simulink model "PartA"  (R2022b)
settings: Solver=VariableStepAuto  StartTime=0.0  StopTime=0.2  RelTol=1e-3
values from neighbouring files (symbols this model uses):
  Freq = 60    [main.mat]    (also in main1.m)
  Lload = 0.01    [main.mat]    (also in main1.m)
  Rload = 2    [main.mat]    (also in main1.m)
  Vdc = 250    [main.mat]    (also in main1.m)
libraries: spspowerguiLib x1
settings Model: Creator=pouyaalaei  LastModifiedBy=igho
settings SolverCC: AlgebraicLoopSolver=TrustRegion
settings DataIOCC: ReturnWorkspaceOutputs=off
settings DebuggingCC: UnconnectedInputMsg=warning  UnconnectedOutputMsg=warning  UnconnectedLineMsg=warning  SFMachineParentedDataDiag=warning
settings ModelReferenceCC: EnableRefExpFcnMdlSchedulingChecks=on
settings RTWCC: DLArmComputeVersion=19.05

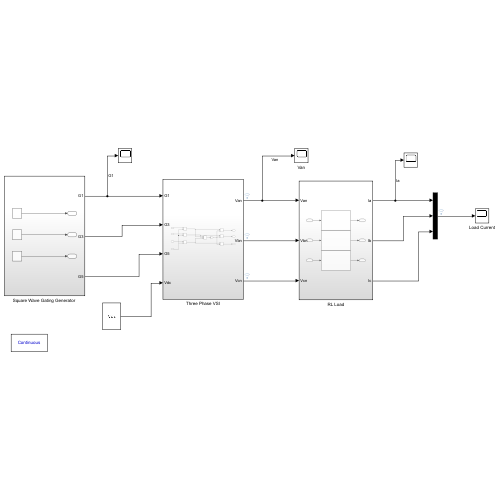
[thumbnail: Simulink's stored preview of the top-level diagram]
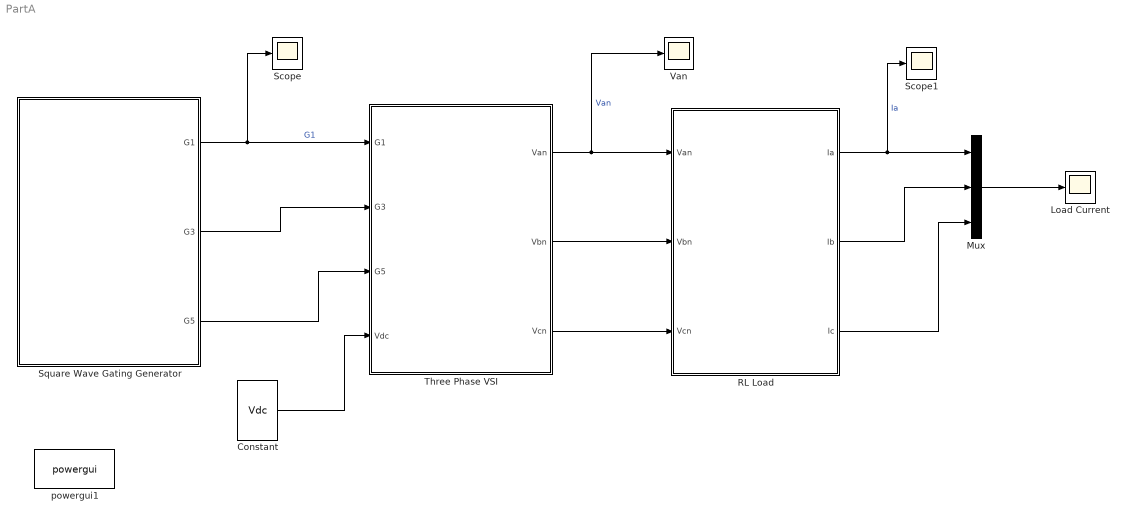
== system PartA ==
  Constant : Constant  Value=Vdc
  Load Current : Scope
  Mux : Mux  Inputs=3
  RL Load : Subsystem
  Scope : Scope
  Scope1 : Scope
  "Square Wave Gating Generator " : Subsystem
  Three Phase VSI : Subsystem
  Van : Scope
  powergui1 : spspowerguiLib/powergui  Priority=1  SimulationMode=Continuous  SampleTime=50e-6  frequency=60  Iterations=50  frequencyindice=60  Pbase=100e6  ErrMax=1e-4  UnitsV=kV  UnitsW=MW  buscounter=0  FunctionMessages=off  echomessages=off  EnableUseOfTLC=off  CurrentSourceSwitches=off  DisableSnubberDevices=off  DisableRonSwitches=off  DisableVfSwitches=off  DisplayEquations=off  AutomaticDiscreteSolvers=off  SolverType=Tustin/Backward Euler (TBE)  Interpol=off  ExternalGateDelay=off  methode=off  Ts=100  x0status=blocks  SPID=on  SwTol=0  HookPort=off  NonlinearTolerance=1e-4  nMaxIteration=100  ContinueOnMaxIteration=off  RestoreLinks=warning  ResistiveCurrentMeasurement=off  Frange=[0:2:500]  Ylog=off  Xlog=on  ShowGrid=off  save=off  variable=ZData  structure=0  ZoomFFT=off  StartTime=0.0  cycles=1  DisplayStyle=1  fundamental=60  FreqAxis=off  MaxFrequency=1000  frequencyindicesteady=1  RmsSteady=1  display=off
  wires:
  "Square Wave Gating Generator "/1(G1) -> Scope/1, Three Phase VSI/1(G1)  "G1"
  "Square Wave Gating Generator "/2(G3) -> Three Phase VSI/2(G3)
  "Square Wave Gating Generator "/3(G5) -> Three Phase VSI/3(G5)
  Constant/1 -> Three Phase VSI/4(Vdc)
  Three Phase VSI/1(Van) -> Van/1, RL Load/1(Van)  "Van"
  Three Phase VSI/2(Vbn) -> RL Load/2(Vbn)
  Three Phase VSI/3(Vcn) -> RL Load/3(Vcn)
  RL Load/1(Ia) -> Scope1/1, Mux/1  "Ia"
  RL Load/2(Ib) -> Mux/2
  RL Load/3(Ic) -> Mux/3
  Mux/1 -> Load Current/1

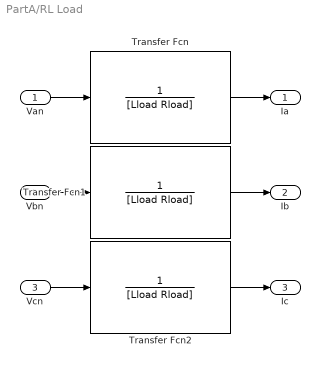
== system PartA/RL Load ==
  Van : Inport
  Vbn : Inport  Port=2
  Vcn : Inport  Port=3
  Transfer Fcn : TransferFcn  Denominator=[Lload Rload]
  Transfer Fcn1 : TransferFcn  Denominator=[Lload Rload]
  Transfer Fcn2 : TransferFcn  Denominator=[Lload Rload]
  Ia : Outport
  Ib : Outport  Port=2
  Ic : Outport  Port=3
  wires:
  Van/1 -> Transfer Fcn/1
  Vbn/1 -> Transfer Fcn1/1
  Vcn/1 -> Transfer Fcn2/1
  Transfer Fcn2/1 -> Ic/1
  Transfer Fcn1/1 -> Ib/1
  Transfer Fcn/1 -> Ia/1

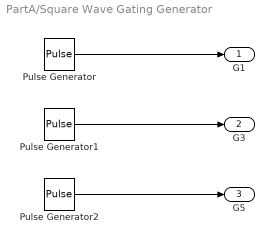
== system PartA/Square Wave Gating Generator  ==
  Pulse Generator : DiscretePulseGenerator  PulseType=Time based  Period=1/Freq  PulseWidth=50
  Pulse Generator1 : DiscretePulseGenerator  PulseType=Time based  Period=1/Freq  PulseWidth=50  PhaseDelay=1/Freq*120/360
  Pulse Generator2 : DiscretePulseGenerator  PulseType=Time based  Period=1/Freq  PulseWidth=50  PhaseDelay=-1/Freq*120/360
  G1 : Outport
  G3 : Outport  Port=2
  G5 : Outport  Port=3
  wires:
  Pulse Generator2/1 -> G5/1
  Pulse Generator1/1 -> G3/1
  Pulse Generator/1 -> G1/1

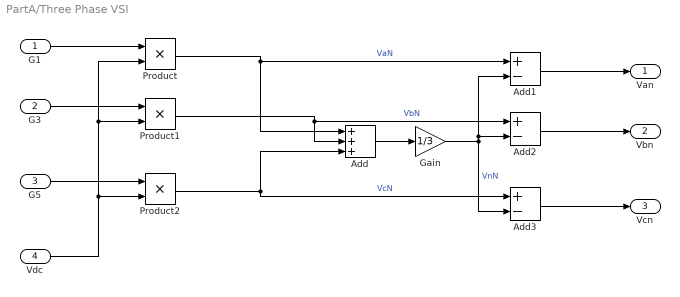
== system PartA/Three Phase VSI ==
  G1 : Inport
  G3 : Inport  Port=2
  G5 : Inport  Port=3
  Vdc : Inport  Port=4
  Add : Sum  Inputs=+++
  Add1 : Sum  Inputs=+-
  Add2 : Sum  Inputs=+-
  Add3 : Sum  Inputs=+-
  Gain : Gain  Gain=1/3
  Product : Product
  Product1 : Product
  Product2 : Product
  Van : Outport
  Vbn : Outport  Port=2
  Vcn : Outport  Port=3
  wires:
  G3/1 -> Product1/1
  G1/1 -> Product/1
  G5/1 -> Product2/1
  Vdc/1 -> Product/2, Product1/2, Product2/2
  Product/1 -> Add1/1, Add/1  "VaN"
  Product1/1 -> Add2/1, Add/2  "VbN"
  Product2/1 -> Add/3, Add3/1  "VcN"
  Add/1 -> Gain/1
  Gain/1 -> Add1/2, Add2/2, Add3/2  "VnN"
  Add1/1 -> Van/1
  Add2/1 -> Vbn/1
  Add3/1 -> Vcn/1
